simulink model "sim123NF"  (Simulink 9.3)
settings: Solver=ode4  StartTime=0.0  StopTime=601  FixedStep=0.001  RelTol=1e-3  EnableMultiTasking=on
values from neighbouring files (symbols this model uses):
  ctrl_idx = strToIdx(actStr,loadNames)    [Driver_oaklandJ_stepresp.m]    (also in driver_runDailySim.m = [make_busOrder(busNames_short,loadNames(ctrl_idx_align(1:len; driver_runMultiple.m = [make_busOrder(busNames_short,loadNames(ctrl_idx_align(1:len)
  dbc_idx = strToIdx(dbcStr,loadNames)    [Driver_oaklandJ_stepresp.m]    (also in driver_runDailySim.m; driver_runMultiple.m)
  Ki_vang = Ki_vang*(1/3)    [Driver_oaklandJ_run.m]    (also in Driver_oaklandJ_stepresp.m = zeros(r,1))
  Ki_vmag = Ki_vmag*(1/3)    [Driver_oaklandJ_run.m]    (also in Driver_oaklandJ_stepresp.m = zeros(r,1))
  Kp_vang = Kp_vang*(1/3)    [Driver_oaklandJ_run.m]    (also in Driver_oaklandJ_stepresp.m = zeros(r,1))
  Kp_vmag = Kp_vmag*(1/3)    [Driver_oaklandJ_run.m]    (also in Driver_oaklandJ_stepresp.m = zeros(r,1))
  meas_idx = strToIdx(measStr,busNames)    [Driver_oaklandJ_stepresp.m]    (also in driver_runDailySim.m; driver_runMultiple.m)
  Options = [1 1]    [Driver_oaklandJ_stepresp.m]    (also in driver_runDailySim.m; driver_runMultiple.m)
  perf_Vbase = V1base    [Driver_oaklandJ_stepresp.m]    (also in driver_runDailySim.m; driver_runMultiple.m)
  RscTable = [rsc_type' capacity']    [Driver_oaklandJ_stepresp.m]    (also in driver_runDailySim.m; driver_runMultiple.m)
  Sbase = (2581.935^2)    (= 6666388.34422)    [computePU.m]
  Sinv = RscTable(i,2)    [Driver_oaklandJ_stepresp.m]    (also in driver_runDailySim.m; driver_runMultiple.m)
  Ts = 1    [Driver_oaklandJ_stepresp.m]    (also in driver_runDailySim.m; driver_runMultiple.m)
  Vang_ctrlStart = (5+dbcDur*2*maxnum_phAct)+ctrl_start_lag    [Driver_oaklandJ_run.m]    (also in Driver_oaklandJ_stepresp.m = 0; driver_runDailySim.m = 0; driver_runMultiple.m = 0)
  vang_init_actual = vang_new(40,:)    [Driver_oaklandJ_run.m]    (also in Driver_oaklandJ_stepresp.m; PlotLocalCtrl_May15.m = [[0:60:(minEnd-minStart)*60]',repmat(vang_new(2,:),minEnd-mi; driver_runDailySim.m; driver_runMultiple.m)
  Vmag_ctrlStart = (5+dbcDur*2*maxnum_phAct)+ctrl_start_lag    [Driver_oaklandJ_run.m]    (also in Driver_oaklandJ_stepresp.m = 0; driver_runDailySim.m = 0; driver_runMultiple.m = 0)
  vmag_init_actual = vmag_new(40,:)    [Driver_oaklandJ_run.m]    (also in Driver_oaklandJ_stepresp.m; PlotLocalCtrl_May15.m = [[0:60:(minEnd-minStart)*60]',repmat(vmag_new(2,:),minEnd-mi; driver_runDailySim.m; driver_runMultiple.m)
undefined symbols (not defined in the file or in its folder): DiscIntNeverNeededParam, pf_P, pf_Q
libraries: opal_lib x2, rtlab x2, rtlab_phasor x1
Description:
  | Model of a simple control system for use iin training.
settings Model: Creator=Paul Baracos  LastModifiedBy=Jaimie
settings SolverCC: AutoInsertRateTranBlk=on
settings DataIOCC: LimitDataPoints=on  SaveOutput=off  SaveTime=off  SignalLoggingName=sigsOut
settings OptimizationCC: BlockReduction=off  BooleanDataType=off  OptimizeBlockIOStorage=off  BufferReuse=off  GlobalBufferReuse=off  ExpressionFolding=off  LocalBlockOutputs=off  InitFltsAndDblsToZero=on  OptimizeDataStoreBuffers=off  BusAssignmentInplaceUpdate=off
settings DebuggingCC: SaveWithParameterizedLinksMsg=none  SignalResolutionControl=TryResolveAllWithWarning  MultiTaskDSMMsg=warning  MultiTaskCondExecSysMsg=none
settings HardwareCC: TargetUnknown=on
settings GRTTargetCC: TargetFcnLib=ansi_tfl_tmw.mat  GeneratePreprocessorConditionals=Disable all

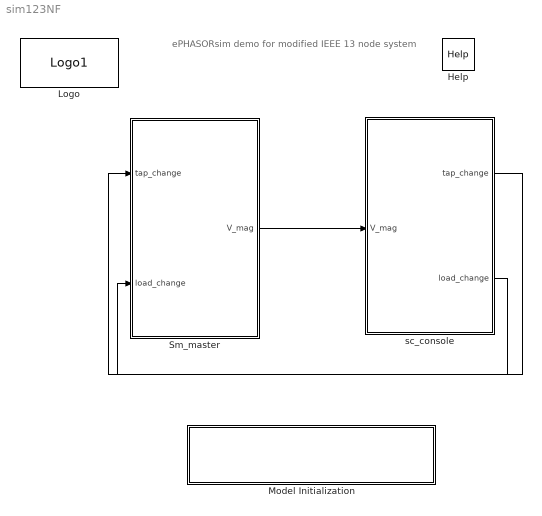
== system sim123NF ==
  note: ePHASORsim demo for
      | modified IEEE 13 node system
  Help : opal_lib/Help  docfile=../help/ePH_IEEE13.html
  Logo : opal_lib/Logo1  vide=[]
  Model Initialization : Subsystem  mask(Model Functions){InitFcnX=, prel=off, posl=off, inif=off, strf=off}
      mask prompts: InitFcnX "Initialisation"; prel "Preload Function"; posl "PostLoad Function"; inif "InitFcn"; strf "StartFcn"
      mask init:
      | currentBlock = gcb;
      | root = bdroot(currentBlock);
      | 
      | if ~strcmp(get_param(root,'BlockDiagramType'),'library')
      |     if prel==1
      |         set_param(root, 'PreLoadFcn', InitFcnX);
      |     else
      |         set_param(root, 'PreLoadFcn', '');
      |     end
      |     if inif==1
      |         set_param(root, 'InitFcn', InitFcnX);
      |     else
      |         set_param(root, 'InitFcn', '');
      |     end
      |     if strf==1
      |         set_param(root, 'StartFcn', InitFcnX);
      |     else
      |         set_param(root, 'StartFcn', '');
      |     end
      |     if posl==1
      |         set_param(root, 'PostLoadFcn', InitFcnX);
      |     else
      |         set_param(root, 'PostLoadFcn', '');
      |     end
      | end
      | 
      | pos = get_param(currentBlock, 'Position');
      | width = pos(3) - pos(1); height = pos(4) - pos(2);
      | txt = [ upper(root) '\n' '- InitFcn. . . . . '  get_param(root, 'InitFcn') ];
      settings: CopyFcn=set_param(gcb,'LinkStatus','none')
      mask Display: text(5, height*0.5, txt, 'horizontalAlignment', 'left', 'verticalAlignment', 'middle') ;
  Sm_master : Subsystem
  sc_console : Subsystem
  wires:
  sc_console/2(load_change) -> Sm_master/2(load_change)
  Sm_master/1(V_mag) -> sc_console/1(V_mag)
  sc_console/1(tap_change) -> Sm_master/1(tap_change)

== system sim123NF/Model Initialization ==

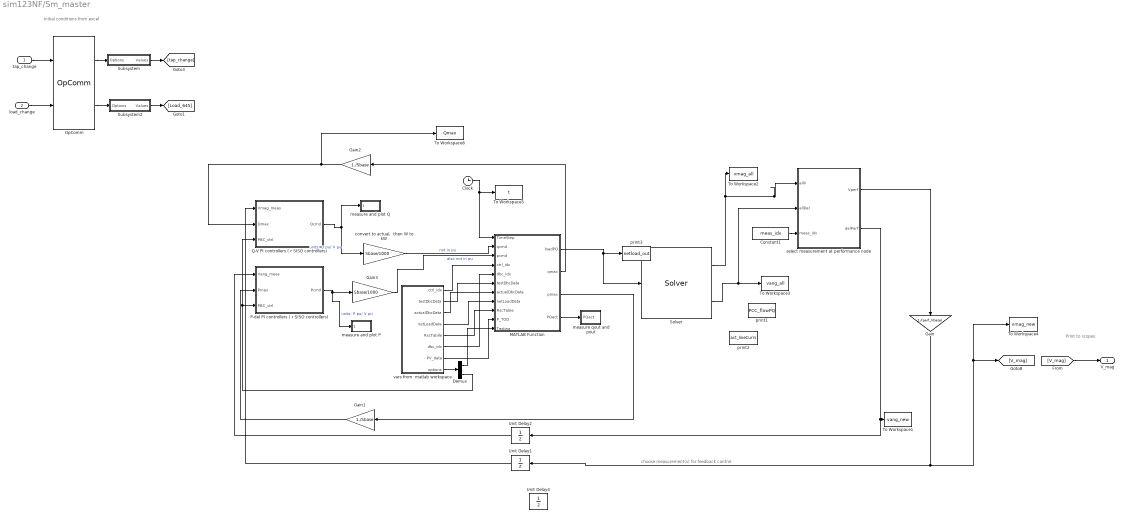
== system sim123NF/Sm_master ==
  note: Initial conditions from excel
  note: choose measurement(s) for feedback control
  note: Print to scopes
  tap_change : Inport
  load_change : Inport  Port=2
  Clock : Clock
  Constant1 : Constant  Value=meas_idx
  Demux : Demux  Outputs=2
  Gain : Gain  Gain=1./(perf_Vbase)
  Gain1 : Gain  Gain=1./Sbase
  Gain2 : Gain  Gain=1./Sbase
  Gain3 : Gain  Gain=Sbase/1000
  MATLAB Function : MATLAB Function  TreatAsAtomicUnit=on
  OpComm : rtlab/OpComm  nbport=2  groupe_acq=1  subsys_rate=0  st=0  Synchronization=on  Interpolation=on  Threshold=1.0  Missed_Data=off  Sim_Time=off  Samples=off  dynSigOut=off  from_console=1  warning_done=off  writeOpCommFile=off  Offset=off
      settings: SourceProductName=RT-LAB
  P-del PI controllers ( r SISO controllers) : Subsystem
  Q-V PI controllers ( r SISO controllers) : Subsystem
  Solver : rtlab_phasor/Solver  epname=System1  extension=Excel  xls='004_GB_IEEE123_OPAL.xlsx'  raw='4992b.raw'  dyr='4992b.dyr'  fmu2builtin=off  cyme='typical.sxst'  cyme_pf=''  cyme_unbalanced=on  powerfactory='network.dgs'  builtin=on  lazy_netlist=off  capidir='CAPI'  fmudir=''  capiprefix=capicomp_  fmuprefix=fmucomp_  logging=off  sim_mode=Power-flow and dynamic simulation  dt=Ts  pf_init_method=Smart Start  pf_tol_v=0.00000001  pf_max_it=100  pf_smart_start=on  pf_flat_start=off  pf_export=on  pfrequest=off  pf_then_dyn=on  np=1  exporty=off  optim_threads=off  perflog_on=off  script_activate_postinit=off  script_postinit_name=''
  Subsystem : Subsystem
  Subsystem2 : Subsystem
  To Workspace1 : ToWorkspace  VariableName=vang_new  SampleTime=Ts
      settings: Save2DSignal=2-D array (concatenate along first dimension)
  To Workspace2 : ToWorkspace  VariableName=vmag_all  SampleTime=Ts
      settings: Save2DSignal=2-D array (concatenate along first dimension)
  To Workspace3 : ToWorkspace  VariableName=vang_all  SampleTime=Ts
      settings: Save2DSignal=2-D array (concatenate along first dimension)
  To Workspace4 : ToWorkspace  VariableName=vmag_new  SampleTime=Ts
      settings: Save2DSignal=2-D array (concatenate along first dimension)
  To Workspace5 : ToWorkspace  VariableName=t  SampleTime=-1
      settings: Save2DSignal=2-D array (concatenate along first dimension)
  To Workspace6 : ToWorkspace  VariableName=Qmax  SampleTime=Ts
  Unit Delay1 : UnitDelay  InitialCondition=vmag_init_actual  SampleTime=Ts  HasFrameUpgradeWarning=on
  Unit Delay2 : UnitDelay  InitialCondition=vang_init_actual  SampleTime=Ts  HasFrameUpgradeWarning=on
  Unit Delay4 : UnitDelay  InitialCondition=vmag_init_actual  SampleTime=Ts  HasFrameUpgradeWarning=on
  "convert to actual,  then W to kW" : Gain  Gain=Sbase/1000
  measure and plot P : Subsystem
  measure and plot Q : Subsystem
  measure qout and pout : Subsystem
  print1 : ToWorkspace  VariableName=PCC_flowPQ  SampleTime=Ts
      settings: Save2DSignal=2-D array (concatenate along first dimension)
  print2 : ToWorkspace  VariableName=act_lineCurrs  SampleTime=Ts
      settings: Save2DSignal=2-D array (concatenate along first dimension)
  print3 : ToWorkspace  VariableName=netload_out  SampleTime=Ts
      settings: Save2DSignal=2-D array (concatenate along first dimension)
  select measurement at performance node : MATLAB Function  TreatAsAtomicUnit=on
  vars from  matlab workspace : Subsystem
  V_mag : Outport
  wires:
  tap_change/1 -> OpComm/1
  load_change/1 -> OpComm/2
  [V_mag] -> V_mag/1
  OpComm/1 -> Subsystem/1(Options)
  OpComm/2 -> Subsystem2/1(Options)
  Subsystem/1(Values) -> [tap_change]
  Subsystem2/1(Values) -> [Load_645]
  vars from  matlab workspace/1("ctrl_idx ") -> MATLAB Function/4(ctrl_idx)
  Constant1/1 -> select measurement at performance node/3(meas_idx)
  vars from  matlab workspace/4(netLoadData) -> MATLAB Function/8(netLoadData)
  Clock/1 -> To Workspace5/1, MATLAB Function/1(TimeStep)
  vars from  matlab workspace/5(RscTablle) -> MATLAB Function/9(RscTable)
  MATLAB Function/2(qmax) -> Gain2/1
  "convert to actual,  then W to kW"/1 -> MATLAB Function/2(qcmd)  "not in pu"
  Gain3/1 -> MATLAB Function/3(pcmd)  "also not in pu"
  vars from  matlab workspace/6(dbc_idx) -> MATLAB Function/5(dbc_idx)
  vars from  matlab workspace/2(testDbcData) -> MATLAB Function/6(testDbcData)
  vars from  matlab workspace/3(actualDbcData) -> MATLAB Function/7(actualDbcData)
  Gain1/1 -> P-del PI controllers ( r SISO controllers)/2(Pmax)
  select measurement at performance node/1(Vperf) -> Gain/1
  Gain2/1 -> Q-V PI controllers ( r SISO controllers)/2(Qmax), To Workspace6/1
  MATLAB Function/3(pmax) -> Gain1/1
  Q-V PI controllers ( r SISO controllers)/1(Qcmd) -> measure and plot Q/1(Qactual), "convert to actual,  then W to kW"/1  "units: Q pu/ V pu"
  P-del PI controllers ( r SISO controllers)/1(Pcmd) -> Gain3/1, measure and plot P/1(Pactual)  "units: P pu/ V pu"
  select measurement at performance node/2(delPerf) -> Unit Delay2/1, To Workspace1/1
  Unit Delay2/1 -> P-del PI controllers ( r SISO controllers)/1(Vang_meas)
  Unit Delay1/1 -> Q-V PI controllers ( r SISO controllers)/1(Vmag_meas)
  MATLAB Function/1(loadPQ) -> print3/1, Solver/1
  Solver/2 -> To Workspace3/1, select measurement at performance node/2(allDel)
  Gain/1 -> Unit Delay1/1, To Workspace4/1, [V_mag]
  Solver/1 -> To Workspace2/1, select measurement at performance node/1(allV)
  vars from  matlab workspace/7(PV_data) -> MATLAB Function/10(P_TOD)
  vars from  matlab workspace/8(options) -> Demux/1
  Demux/1 -> MATLAB Function/11(Testing)
  Demux/2 -> P-del PI controllers ( r SISO controllers)/3(PBC_ctrl), Q-V PI controllers ( r SISO controllers)/3(PBC_ctrl)
  MATLAB Function/4(PQact) -> measure qout and pout/1(PQact)
  ? -> print1/1
  ? -> print2/1

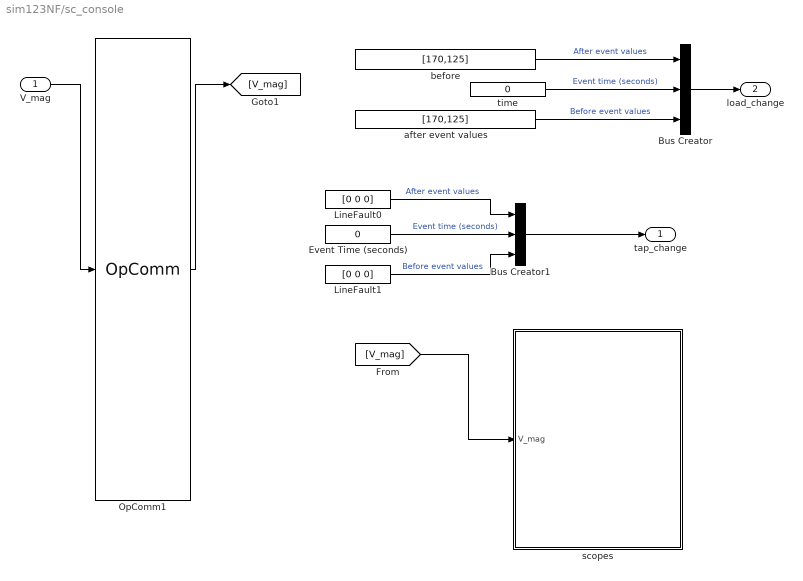
== system sim123NF/sc_console ==
  V_mag : Inport
  Bus Creator : BusCreator  Inputs=3
  Bus Creator1 : BusCreator  Inputs=3
  Event Time (seconds) : Constant  Value=0
  LineFault0 : Constant  Value=[0 0 0]
  LineFault1 : Constant  Value=[0 0 0]
  OpComm1 : rtlab/OpComm  nbport=1  groupe_acq=1  subsys_rate=Ts  st=0  Synchronization=on  Interpolation=on  Threshold=1.0  Missed_Data=off  Sim_Time=off  Samples=off  dynSigOut=off  from_console=0  warning_done=off  writeOpCommFile=off  Offset=off
      settings: SourceProductName=RT-LAB
  after event values : Constant  Value=[170,125]
  before : Constant  Value=[170,125]
  scopes : Subsystem
  time : Constant  Value=0
  tap_change : Outport
  load_change : Outport  Port=2
  wires:
  V_mag/1 -> OpComm1/1
  OpComm1/1 -> [V_mag]
  time/1 -> Bus Creator/2  "Event time (seconds)"
  Bus Creator/1 -> load_change/1
  LineFault0/1 -> Bus Creator1/1  "After event values"
  LineFault1/1 -> Bus Creator1/3  "Before event values"
  Event Time (seconds)/1 -> Bus Creator1/2  "Event time (seconds)"
  Bus Creator1/1 -> tap_change/1
  before/1 -> Bus Creator/1  "After event values"
  after event values/1 -> Bus Creator/3  "Before event values"
  [V_mag] -> scopes/1(V_mag)

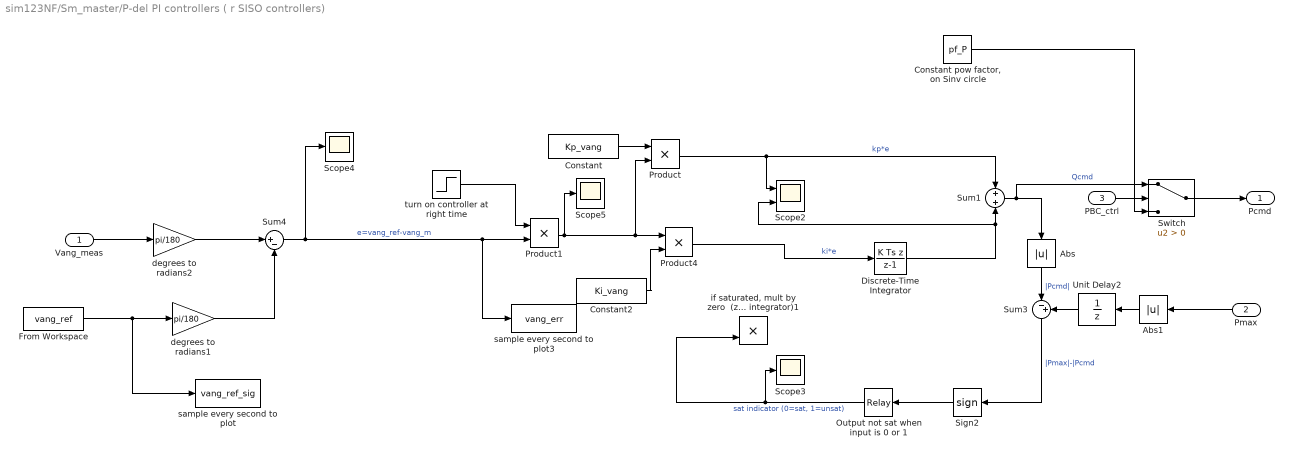
== system sim123NF/Sm_master/P-del PI controllers ( r SISO controllers) ==
  Vang_meas : Inport
  Pmax : Inport  Port=2
  PBC_ctrl : Inport  Port=3
  Abs : Abs
  Abs1 : Abs
  Constant : Constant  Value=Kp_vang
  "Constant pow factor, on Sinv circle" : Constant  Value=pf_P
  Constant2 : Constant  Value=Ki_vang
  Discrete-Time Integrator : DiscreteIntegrator  IntegratorMethod=Integration: Backward Euler  gainval=1  SampleTime=Ts  ICPrevOutput=DiscIntNeverNeededParam  ICPrevScaledInput=DiscIntNeverNeededParam
  From Workspace : FromWorkspace  VariableName=vang_ref  SampleTime=0
  "Output not sat when input is 0 or 1 " : Relay  OnSwitchValue=-0.5  OffSwitchValue=-0.5
  Product : Product
  Product1 : Product
  Product4 : Product
  Scope2 : Scope  NumInputPorts=2
  Scope3 : Scope
  Scope4 : Scope
  Scope5 : Scope
  Sign2 : Signum
  Sum1 : Sum  Inputs=+|+
  Sum3 : Sum  Inputs=|-+
  Sum4 : Sum  Inputs=|+-
  Switch : Switch  Criteria=u2 > Threshold
  Unit Delay2 : UnitDelay  InitialCondition=Sinv*ones(size(Kp_vang))  SampleTime=Ts  HasFrameUpgradeWarning=on
  degrees to radians1 : Gain  Gain=pi/180
  degrees to radians2 : Gain  Gain=pi/180
  "if saturated, mult by zero  (zero out integrator)1" : Product
  sample every second to plot : ToWorkspace  VariableName=vang_ref_sig  SampleTime=Ts
  sample every second to plot3 : ToWorkspace  VariableName=vang_err  SampleTime=Ts
  turn on controller at right time : Step  Time=Vang_ctrlStart  SampleTime=0
  Pcmd : Outport
  wires:
  Sum4/1 -> sample every second to plot3/1, Product1/2, Scope4/1  "e=vang_ref-vang_m"
  Constant/1 -> Product/1
  turn on controller at right time/1 -> Product1/1
  Product1/1 -> Product/2, Product4/1, Scope5/1
  Constant2/1 -> Product4/2
  Product/1 -> Scope2/1, Sum1/1  "kp*e"
  Sum3/1 -> Sign2/1  "|Pmax|-|Pcmd"
  Product4/1 -> Discrete-Time Integrator/1  "ki*e"
  Pmax/1 -> Abs1/1
  Abs/1 -> Sum3/1  "|Pcmd|"
  "Output not sat when input is 0 or 1 "/1 -> Scope3/1, "if saturated, mult by zero  (zero out integrator)1"/2  "sat indicator (0=sat, 1=unsat)"
  Discrete-Time Integrator/1 -> Scope2/2, Sum1/2
  Unit Delay2/1 -> Sum3/2
  Abs1/1 -> Unit Delay2/1
  Vang_meas/1 -> degrees to radians2/1
  From Workspace/1 -> sample every second to plot/1, degrees to radians1/1
  Sign2/1 -> "Output not sat when input is 0 or 1 "/1
  Sum1/1 -> Switch/1, Abs/1  "Qcmd"
  "Constant pow factor, on Sinv circle"/1 -> Switch/3
  PBC_ctrl/1 -> Switch/2
  Switch/1 -> Pcmd/1
  degrees to radians2/1 -> Sum4/1
  degrees to radians1/1 -> Sum4/2

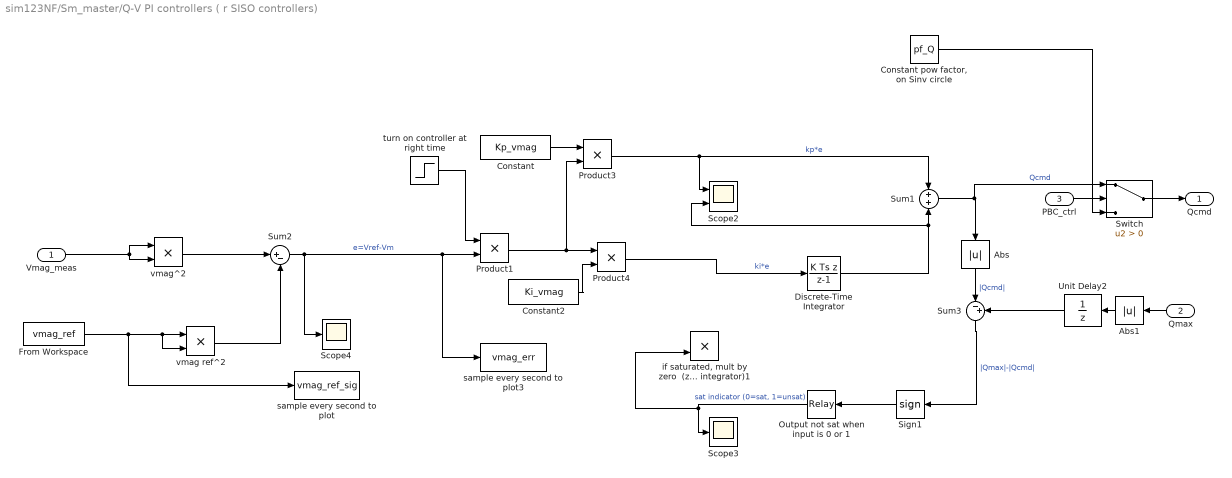
== system sim123NF/Sm_master/Q-V PI controllers ( r SISO controllers) ==
  Vmag_meas : Inport
  Qmax : Inport  Port=2
  PBC_ctrl : Inport  Port=3
  Abs : Abs
  Abs1 : Abs
  Constant : Constant  Value=Kp_vmag
  "Constant pow factor, on Sinv circle" : Constant  Value=pf_Q
  Constant2 : Constant  Value=Ki_vmag
  Discrete-Time Integrator : DiscreteIntegrator  IntegratorMethod=Integration: Backward Euler  gainval=1  SampleTime=Ts  ICPrevOutput=DiscIntNeverNeededParam  ICPrevScaledInput=DiscIntNeverNeededParam
  From Workspace : FromWorkspace  VariableName=vmag_ref  SampleTime=0
  Output not sat when input is 0 or 1 : Relay  OnSwitchValue=-0.5  OffSwitchValue=-0.5
  Product1 : Product
  Product3 : Product
  Product4 : Product
  Scope2 : Scope  NumInputPorts=2
  Scope3 : Scope
  Scope4 : Scope
  Sign1 : Signum
  Sum1 : Sum  Inputs=+|+
  Sum2 : Sum  Inputs=|+-
  Sum3 : Sum  Inputs=|-+
  Switch : Switch  Criteria=u2 > Threshold
  Unit Delay2 : UnitDelay  InitialCondition=Sinv*ones(size(Kp_vmag))  SampleTime=Ts  HasFrameUpgradeWarning=on
  "if saturated, mult by zero  (zero out integrator)1" : Product
  sample every second to plot : ToWorkspace  VariableName=vmag_ref_sig  SampleTime=Ts
  sample every second to plot3 : ToWorkspace  VariableName=vmag_err  SampleTime=Ts
  turn on controller at right time : Step  Time=Vmag_ctrlStart  SampleTime=0
  vmag ref^2 : Product
  vmag^2 : Product
  Qcmd : Outport
  wires:
  Sum2/1 -> sample every second to plot3/1, Product1/2, Scope4/1  "e=Vref-Vm"
  Constant/1 -> Product3/1
  turn on controller at right time/1 -> Product1/1
  Product1/1 -> Product4/1, Product3/2
  Constant2/1 -> Product4/2
  Product3/1 -> Scope2/1, Sum1/1  "kp*e"
  Sum1/1 -> Switch/1, Abs/1  "Qcmd"
  Sum3/1 -> Sign1/1  "|Qmax|-|Qcmd|"
  Product4/1 -> Discrete-Time Integrator/1  "ki*e"
  Qmax/1 -> Abs1/1
  Abs/1 -> Sum3/1  "|Qcmd|"
  Output not sat when input is 0 or 1/1 -> Scope3/1, "if saturated, mult by zero  (zero out integrator)1"/2  "sat indicator (0=sat, 1=unsat)"
  Discrete-Time Integrator/1 -> Scope2/2, Sum1/2
  Unit Delay2/1 -> Sum3/2
  Abs1/1 -> Unit Delay2/1
  From Workspace/1 -> vmag ref^2/2, vmag ref^2/1, sample every second to plot/1
  Sign1/1 -> Output not sat when input is 0 or 1/1
  PBC_ctrl/1 -> Switch/2
  Switch/1 -> Qcmd/1
  "Constant pow factor, on Sinv circle"/1 -> Switch/3
  Vmag_meas/1 -> vmag^2/1, vmag^2/2
  vmag^2/1 -> Sum2/1
  vmag ref^2/1 -> Sum2/2

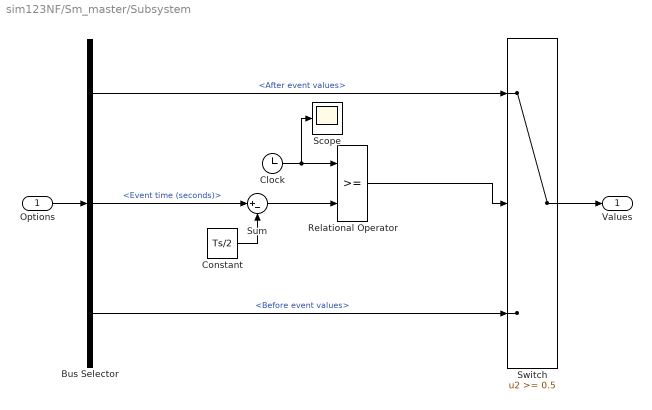
== system sim123NF/Sm_master/Subsystem ==
  Options : Inport
  Bus Selector : BusSelector  OutputSignals=After event values,Event time (seconds),Before event values
  Clock : Clock
  Constant : Constant  Value=Ts/2
  Relational Operator : RelationalOperator  OutDataTypeStr=boolean  RndMeth=Nearest
  Scope : Scope
  Sum : Sum  Inputs=|+-
  Switch : Switch  Threshold=0.5
  Values : Outport
  wires:
  Clock/1 -> Scope/1, Relational Operator/1
  Constant/1 -> Sum/2
  Sum/1 -> Relational Operator/2
  Bus Selector/2 -> Sum/1  "<Event time (seconds)>"
  Relational Operator/1 -> Switch/2
  Bus Selector/3 -> Switch/3  "<Before event values>"
  Bus Selector/1 -> Switch/1  "<After event values>"
  Switch/1 -> Values/1
  Options/1 -> Bus Selector/1

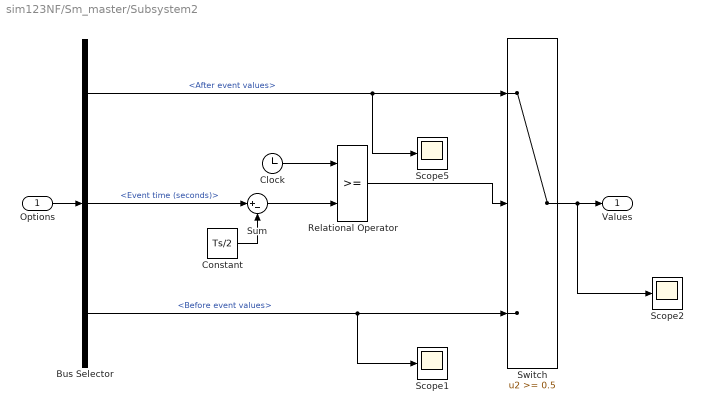
== system sim123NF/Sm_master/Subsystem2 ==
  Options : Inport
  Bus Selector : BusSelector  OutputSignals=After event values,Event time (seconds),Before event values
  Clock : Clock
  Constant : Constant  Value=Ts/2
  Relational Operator : RelationalOperator  OutDataTypeStr=boolean  RndMeth=Nearest
  Scope1 : Scope
  Scope2 : Scope
  Scope5 : Scope
  Sum : Sum  Inputs=|+-
  Switch : Switch  Threshold=0.5
  Values : Outport
  wires:
  Clock/1 -> Relational Operator/1
  Constant/1 -> Sum/2
  Sum/1 -> Relational Operator/2
  Bus Selector/2 -> Sum/1  "<Event time (seconds)>"
  Relational Operator/1 -> Switch/2
  Bus Selector/3 -> Switch/3, Scope1/1  "<Before event values>"
  Bus Selector/1 -> Switch/1, Scope5/1  "<After event values>"
  Switch/1 -> Values/1, Scope2/1
  Options/1 -> Bus Selector/1

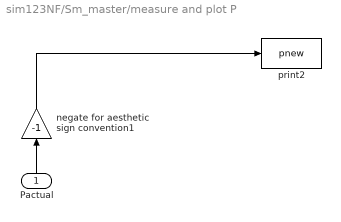
== system sim123NF/Sm_master/measure and plot P ==
  Pactual : Inport
  negate for aesthetic  sign convention1 : Gain  Gain=-1
  print2 : ToWorkspace  VariableName=pnew  SampleTime=Ts
      settings: Save2DSignal=2-D array (concatenate along first dimension)
  wires:
  Pactual/1 -> negate for aesthetic  sign convention1/1
  negate for aesthetic  sign convention1/1 -> print2/1

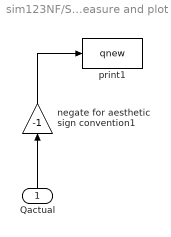
== system sim123NF/Sm_master/measure and plot Q ==
  Qactual : Inport
  negate for aesthetic  sign convention1 : Gain  Gain=-1
  print1 : ToWorkspace  VariableName=qnew  SampleTime=Ts
      settings: Save2DSignal=2-D array (concatenate along first dimension)
  wires:
  Qactual/1 -> negate for aesthetic  sign convention1/1
  negate for aesthetic  sign convention1/1 -> print1/1

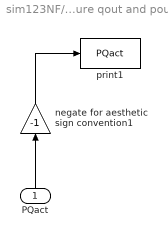
== system sim123NF/Sm_master/measure qout and pout ==
  PQact : Inport
  negate for aesthetic  sign convention1 : Gain  Gain=-1
  print1 : ToWorkspace  VariableName=PQact  SampleTime=Ts
      settings: Save2DSignal=2-D array (concatenate along first dimension)
  wires:
  PQact/1 -> negate for aesthetic  sign convention1/1
  negate for aesthetic  sign convention1/1 -> print1/1

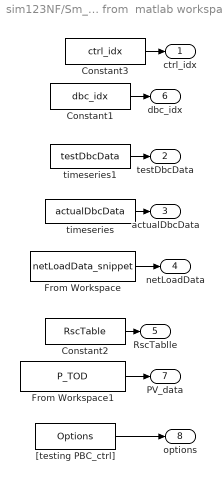
== system sim123NF/Sm_master/vars from  matlab workspace ==
  Constant1 : Constant  Value=dbc_idx
  Constant2 : Constant  Value=RscTable
  Constant3 : Constant  Value=ctrl_idx
  From Workspace : FromWorkspace  VariableName=netLoadData_snippet  OutDataTypeStr=double  SampleTime=Ts  Interpolate=off  OutputAfterFinalValue=Setting to zero
  From Workspace1 : FromWorkspace  VariableName=P_TOD  OutDataTypeStr=double  SampleTime=Ts  Interpolate=off  OutputAfterFinalValue=Holding final value
  "[testing PBC_ctrl]" : Constant  Value=Options
  timeseries : FromWorkspace  VariableName=actualDbcData  SampleTime=Ts  Interpolate=off  OutputAfterFinalValue=Holding final value
  timeseries1 : FromWorkspace  VariableName=testDbcData  OutDataTypeStr=double  SampleTime=Ts  Interpolate=off  OutputAfterFinalValue=Holding final value
  "ctrl_idx " : Outport
  testDbcData : Outport  Port=2
  actualDbcData : Outport  Port=3
  netLoadData : Outport  Port=4
  RscTablle : Outport  Port=5
  dbc_idx : Outport  Port=6
  PV_data : Outport  Port=7
  options : Outport  Port=8
  wires:
  Constant1/1 -> dbc_idx/1
  From Workspace/1 -> netLoadData/1
  timeseries1/1 -> testDbcData/1
  timeseries/1 -> actualDbcData/1
  Constant2/1 -> RscTablle/1
  From Workspace1/1 -> PV_data/1
  Constant3/1 -> "ctrl_idx "/1
  "[testing PBC_ctrl]"/1 -> options/1

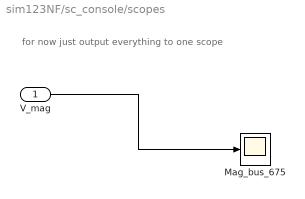
== system sim123NF/sc_console/scopes ==
  note: for now just output everything to one scope
  V_mag : Inport
  Mag_bus_675 : Scope
  wires:
  V_mag/1 -> Mag_bus_675/1

== matlab function Sm_master/select measurement at performance node ==
  data: Vperf output double; allV input double; allDel input double; delPerf output double; meas_idx input double
function [Vperf,delPerf]=selectMeas(allV,allDel,meas_idx)
% use measStr,nodeNames from workspace
    Vperf=allV(meas_idx);
    delPerf=allDel(meas_idx);
end

== matlab function Sm_master/MATLAB Function ==
  data: TimeStep input double; qcmd input double; pcmd input double; loadPQ output double size=236; qmax output double; ctrl_idx input double; dbc_idx input double; testDbcData input double; actualDbcData input double; netLoadData input double size=236; RscTable input double; pmax output double; PQact output double; P_TOD input double; Testing input double
function [loadPQ, qmax ,pmax, PQact]  = updatePows(TimeStep,qcmd,pcmd,ctrl_idx,dbc_idx,testDbcData,actualDbcData,netLoadData,RscTable,P_TOD,Testing)
% netLoadData, dbcData, and k are timeseries, fed once by one for each timestep
% ctrl_idx and dbc_idx are constant
    % inputs: 
        % k is current timestep
        % 3x1 vectors of unadjusted actuation, as if have 1 actuator and it's located at the perf node 
    % inputs: rx1 vectors of powers at all nodes 
        % r is number of phases across all nodes, i.e. the dim of the pin
        % vector input to RTlab solve
%      TimeStep  % in seconds

    % for testdbc uncontrolled sim dont wany any limits
    pout=pcmd; pout=pout(:); qout=qcmd; qout=qout(:); % make column vectors
    pmax=10000*ones(size(pcmd)); qmax=10000*ones(size(pcmd)); % 
    
    alpha=0.85; %inverter bit oversized for PC
    % for controlled sim apply resource constraints
    if ~Testing % if not doing step response tests
        allSinv=RscTable(:,2); % column vec of all capacity values
        pmax=allSinv; 

        for i=1:size(RscTable,1) % for each phase-actuator
            Sinv=RscTable(i,2);
            type=RscTable(i,1);
            switch type
                case 1 % battery+PV, 4 quad op wrt P_TOD
                    pmax(i)=min( [alpha*Sinv,P_TOD(i)] ); % up to P_TOD, and in direction of pcmd
                case 2 % EV,4 quad op
                    pmax(i)=alpha*Sinv; 
                case 3 % battery only, 4 quad op
                    pmax(i)=alpha*Sinv; 
                otherwise
                    error('did not recognize resource type');
            end
            
            if pmax(i)<=Sinv
                qmax(i)=sqrt(Sinv^2-pmax(i)^2);
            else
                qmax(i)=0;
            end
            qout(i)=sign(qcmd(i)) * min(qmax(i),abs(qcmd(i)));
            pout(i)=sign(pcmd(i)) * min(pmax(i),abs(pcmd(i)));

        end
    end

    %% assign outputs: [loadPQ, qmax ,pmax, PQact]

    actpq=[pout qout]; % P in first col, Q in second
    PQact = reshape(actpq,[1,length(ctrl_idx)]).'; % make col vec with Ps grouped then Qs grouped
    a=reshape(testDbcData,[2,length(ctrl_idx)/2]);
    testDbcData=reshape(a',[length(ctrl_idx),1]); % make col vec with Ps grouped then Qs grouped
    a=reshape(actualDbcData,[2,length(dbc_idx)/2]);
    actualDbcData=reshape(a',[length(dbc_idx),1]); % make col vec with Ps grouped then Qs grouped

    loadPQ=netLoadData; % P&Q, ordered according to loadNames
%    if (TimeStep<5 && TimeStep>3) % in seconds
%         loadPQ(ctrl_idx)+PQact+testDbcData
%     end
    loadPQ(ctrl_idx)=loadPQ(ctrl_idx)+PQact+testDbcData;
    loadPQ(dbc_idx)=loadPQ(dbc_idx)+actualDbcData;

end
